simulink model "Lab2_3_sol"  (R2015b)
settings: Solver=VariableStepDiscrete  StartTime=0.0  StopTime=256*256*2  RelTol=1e-3
PreLoadFcn:
  | ImSize = 256;
undefined symbols (not defined in the file): gray
libraries: xbsIndex_r4 x32, dspsigattribs x5, visionsinks x2, visionsources x1
settings Model: Creator=arvinds  LastModifiedBy=duncanm
settings DataIOCC: SaveFormat=Array  SignalLoggingSaveFormat=ModelDataLogs
settings OptimizationCC: ExpressionDepthLimit=2147483647
settings DebuggingCC: UnderspecifiedInitializationDetection=Classic  MergeDetectMultiDrivingBlocksExec=none  SolverPrmCheckMsg=warning  FcnCallInpInsideContextMsg=EnableAllAsWarning  StateNameClashWarn=warning
settings HardwareCC: ProdBitPerPointer=32  ProdLargestAtomicFloat=None  ProdIntDivRoundTo=Undefined  ProdEndianess=Unspecified  ProdWordSize=32  ProdHWDeviceType=32-bit Generic
settings GRTTargetCC: GeneratePreprocessorConditionals=Disable all  CombineOutputUpdateFcns=off  GRTInterface=on
settings ConfigComp: CovModelRefEnable=Off  CovSFcnEnable=off

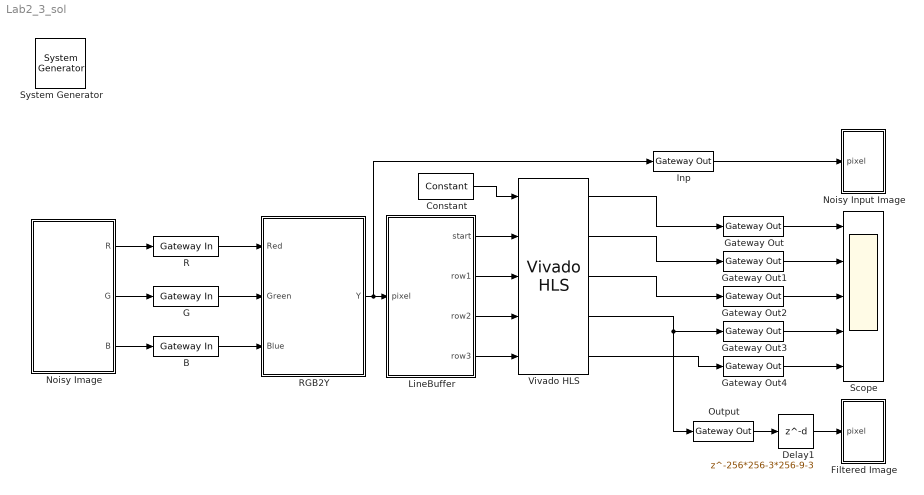
== system Lab2_3_sol ==
  " System Generator" : xbsIndex_r4/ System Generator  Tag=genX  xilinxfamily=kintex7  part=xc7k325t  speed=-3  package=fbg676  synthesis_tool=Vivado  clock_wrapper=Clock Enables  directory=./netlist  proj_type=Project Navigator  Synth_file=XST Defaults  Impl_file=ISE Defaults  testbench=off  simulink_period=1  sysclk_period=5  dcm_input_clock_period=10  incr_netlist=off  trim_vbits=Everywhere in SubSystem  dbl_ovrd=According to Block Masks  core_generation=According to Block Masks  run_coregen=off  deprecated_control=off  eval_field=0  block_type=sysgen
      settings: block_version=14.2
  B : xbsIndex_r4/Gateway In  gui_display_data_type=Fixed-point  arith_type=Unsigned  n_bits=8  bin_pt=0  preci_type=Single  exp_width=8  frac_width=24  rows=1  columns=1  quantization="Round  (unbiased: +/- Inf)"  overflow=Saturate  period=1  UseAsADC=off  ADCChannel='1'  interface=None  automatic_assignment=on  address_offset=hex2dec('00')  intf_name=''  intf_description=''  default_value=0  timing_constraint=None  locs_specified=off  LOCs={}  io_standard={}  inherit_from_input=off  hdl_port=on  dbl_ovrd=off  block_type=gatewayin
      settings: block_version=14.2
  Constant : xbsIndex_r4/Constant  const=0  gui_display_data_type=Boolean  arith_type=Boolean  n_bits=16  bin_pt=14  preci_type=Single  exp_width=8  frac_width=24  explicit_period=off  period=1  equ=P=C  opselect=C  inp2=PCIN>>17  opr=+  inp1=P  carry=CIN  dbl_ovrd=off  block_type=constant
  Delay1 : Delay  DelayLength=256*256-3*256-9-3  SampleTime=1
  Filtered Image : Subsystem
  G : xbsIndex_r4/Gateway In  gui_display_data_type=Fixed-point  arith_type=Unsigned  n_bits=8  bin_pt=0  preci_type=Single  exp_width=8  frac_width=24  rows=1  columns=1  quantization="Round  (unbiased: +/- Inf)"  overflow=Saturate  period=1  UseAsADC=off  ADCChannel='1'  interface=None  automatic_assignment=on  address_offset=hex2dec('00')  intf_name=''  intf_description=''  default_value=0  timing_constraint=None  locs_specified=off  LOCs={}  io_standard={}  inherit_from_input=off  hdl_port=on  dbl_ovrd=off  block_type=gatewayin
      settings: block_version=14.2
  Gateway Out{,1..4} (5 alike) : xbsIndex_r4/Gateway Out  inherit_from_input=off  hdl_port=on  rows=1  columns=1  UseAsDAC=off  DACChannel='1'  interface=None  automatic_assignment=on  address_offset=hex2dec('00')  intf_name=''  intf_description=''  timing_constraint=None  locs_specified=off  LOCs={}  io_standard={}  block_type=gatewayout
  Inp : xbsIndex_r4/Gateway Out  inherit_from_input=on  hdl_port=off  rows=1  columns=1  UseAsDAC=off  DACChannel='1'  interface=None  automatic_assignment=on  address_offset=hex2dec('00')  intf_name=''  intf_description=''  timing_constraint=None  locs_specified=off  LOCs={}  io_standard={}  block_type=gatewayout
      settings: block_version=14.2
  LineBuffer : Subsystem
  Noisy Image : Subsystem
  Noisy Input Image : Subsystem
  Output : xbsIndex_r4/Gateway Out  inherit_from_input=on  hdl_port=on  rows=1  columns=1  UseAsDAC=off  DACChannel='1'  interface=None  automatic_assignment=on  address_offset=hex2dec('00')  intf_name=''  intf_description=''  timing_constraint=None  locs_specified=off  LOCs={}  io_standard={}  block_type=gatewayout
      settings: block_version=14.2
  R : xbsIndex_r4/Gateway In  gui_display_data_type=Fixed-point  arith_type=Unsigned  n_bits=8  bin_pt=0  preci_type=Single  exp_width=8  frac_width=24  rows=1  columns=1  quantization="Round  (unbiased: +/- Inf)"  overflow=Saturate  period=1  UseAsADC=off  ADCChannel='1'  interface=None  automatic_assignment=on  address_offset=hex2dec('00')  intf_name=''  intf_description=''  default_value=0  timing_constraint=None  locs_specified=off  LOCs={}  io_standard={}  inherit_from_input=off  hdl_port=on  dbl_ovrd=off  block_type=gatewayin
      settings: block_version=14.2
  RGB2Y : Subsystem
  Scope : Scope  NumInputPorts=5
  Vivado HLS : xbsIndex_r4/Vivado HLS  anytable='C:/SysGen_Tutorial/Lab7/hls_project/solution1'  fast_sim=off  display_datatype=off  rate_propagation_method=Simulink system period  model_file_path=''  latency=1  block_type=hls
      settings: infoedit=This block allows including C,C++ and SystemC source files in System Generator for DSP designs.
  wires:
  Noisy Image/2(G) -> G/1
  Noisy Image/3(B) -> B/1
  R/1 -> RGB2Y/1(Red)
  G/1 -> RGB2Y/2(Green)
  B/1 -> RGB2Y/3(Blue)
  RGB2Y/1(Y) -> LineBuffer/1(pixel), Inp/1
  LineBuffer/2(row1) -> Vivado HLS/3
  LineBuffer/3(row2) -> Vivado HLS/4
  LineBuffer/4(row3) -> Vivado HLS/5
  Noisy Image/1(R) -> R/1
  Output/1 -> Delay1/1
  Inp/1 -> Noisy Input Image/1(pixel)
  Delay1/1 -> Filtered Image/1(pixel)
  Vivado HLS/4 -> Output/1, Gateway Out3/1
  Vivado HLS/1 -> Gateway Out/1
  Vivado HLS/2 -> Gateway Out1/1
  Vivado HLS/3 -> Gateway Out2/1
  Vivado HLS/5 -> Gateway Out4/1
  Gateway Out/1 -> Scope/1
  Gateway Out1/1 -> Scope/2
  Gateway Out2/1 -> Scope/3
  Gateway Out3/1 -> Scope/4
  Gateway Out4/1 -> Scope/5
  LineBuffer/1(start) -> Vivado HLS/2
  Constant/1 -> Vivado HLS/1

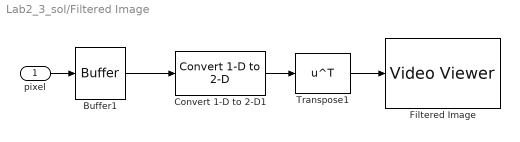
== system Lab2_3_sol/Filtered Image ==
  pixel : Inport
  Buffer1 : Buffer  N=ImSize*ImSize  TreatMby1Signals=One channel
  Convert 1-D to 2-D1 : dspsigattribs/Convert 1-D to 2-D  M=ImSize  N=ImSize  frameBasedOut=off
  Filtered Image : visionsinks/Video Viewer  inputType=Obsolete7b  imagePorts=One multidimensional signal  useColorMap=off  colormapValue=gray(256)  specRange=off  minInputVal=0  maxInputVal=255  FigPos=[721 702.8 408 300]  AxisZoom=on  trueSizedOnce=off  OpenAtMdlStart=on  DefaultConfigurationName=vipscopes.VideoViewerScopeCfg
  Transpose1 : Math  Operator=transpose  SaturateOnIntegerOverflow=on
  wires:
  Buffer1/1 -> Convert 1-D to 2-D1/1
  Convert 1-D to 2-D1/1 -> Transpose1/1
  pixel/1 -> Buffer1/1
  Transpose1/1 -> Filtered Image/1

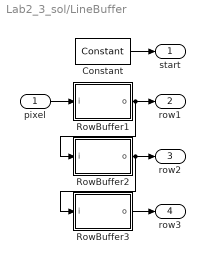
== system Lab2_3_sol/LineBuffer ==
  pixel : Inport
  Constant : xbsIndex_r4/Constant  const=1  gui_display_data_type=Boolean  arith_type=Boolean  n_bits=16  bin_pt=14  preci_type=Single  exp_width=8  frac_width=24  explicit_period=off  period=1  equ=P=C  opselect=C  inp2=PCIN>>17  opr=+  inp1=P  carry=CIN  dbl_ovrd=off  block_type=constant
  RowBuffer1 : Subsystem  mask(Virtex2 Line Buffer){buf_depth=ImSize, cst=1}
      mask prompts: buf_depth "Buffer Depth"; cst "Sample Period"
      mask help: The Xilinx Virtex2 Line Buffer reference block delayes a sequential stream of pixels by the specified buffer depth. It is optimized for the Virtex2 family since it uses the Read Before Write option on the underlying Single Port RAM block.
      mask init:
      | str = sprintf('-%d',buf_depth);
      | [bg,fg] = xlcmap('XBlock',0);
      | iPos = get_param(gcb,'Position');
      | iWidth=iPos(3)-iPos(1); iHeight=iPos(4)-iPos(2);
      | iCx=iWidth/2;
      | iCy=iHeight/2;
      | [logoX, logoY] = xlogo(iPos);
      mask Help: eval('');xlDoc('-book','sysgen','-topic','Virtex2_Line_Buffer');
      mask Display:
      | patch([0 iWidth iWidth 0],[0 0 iHeight iHeight] , bg);
      | patch(logoX,logoY , fg);
      | text(iCx-6,iCy,'z');
      | text(iCx,iCy+4,str);
      | plot([0 0 iWidth iWidth 0], [0 iHeight iHeight 0 0]);
  RowBuffer2 : Subsystem  mask(Virtex2 Line Buffer){buf_depth=ImSize, cst=1}
      mask prompts: buf_depth "Buffer Depth"; cst "Sample Period"
      mask help: The Xilinx Virtex2 Line Buffer reference block delayes a sequential stream of pixels by the specified buffer depth. It is optimized for the Virtex2 family since it uses the Read Before Write option on the underlying Single Port RAM block.
      mask init: same as Lab2_3_sol/LineBuffer/RowBuffer1
      mask Help: eval('');xlDoc('-book','sysgen','-topic','Virtex2_Line_Buffer');
      mask Display:
      | patch([0 iWidth iWidth 0],[0 0 iHeight iHeight] , bg);
      | patch(logoX,logoY , fg);
      | text(iCx-6,iCy,'z');
      | text(iCx,iCy+4,str);
      | plot([0 0 iWidth iWidth 0], [0 iHeight iHeight 0 0]);
  RowBuffer3 : Subsystem  mask(Virtex2 Line Buffer){buf_depth=ImSize, cst=1}
      mask prompts: buf_depth "Buffer Depth"; cst "Sample Period"
      mask help: The Xilinx Virtex2 Line Buffer reference block delayes a sequential stream of pixels by the specified buffer depth. It is optimized for the Virtex2 family since it uses the Read Before Write option on the underlying Single Port RAM block.
      mask init: same as Lab2_3_sol/LineBuffer/RowBuffer1
      mask Help: eval('');xlDoc('-book','sysgen','-topic','Virtex2_Line_Buffer');
      mask Display:
      | patch([0 iWidth iWidth 0],[0 0 iHeight iHeight] , bg);
      | patch(logoX,logoY , fg);
      | text(iCx-6,iCy,'z');
      | text(iCx,iCy+4,str);
      | plot([0 0 iWidth iWidth 0], [0 iHeight iHeight 0 0]);
  start : Outport
  row1 : Outport  Port=2
  row2 : Outport  Port=3
  row3 : Outport  Port=4
  wires:
  RowBuffer1/1(o) -> RowBuffer2/1(i), row1/1
  RowBuffer2/1(o) -> RowBuffer3/1(i), row2/1
  pixel/1 -> RowBuffer1/1(i)
  RowBuffer3/1(o) -> row3/1
  Constant/1 -> start/1

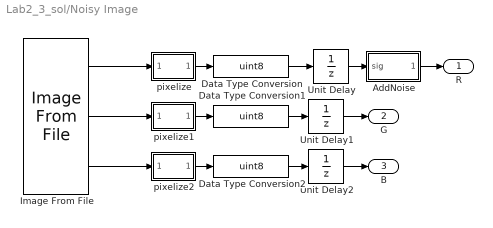
== system Lab2_3_sol/Noisy Image ==
  AddNoise : Subsystem
  Data Type Conversion : DataTypeConversion  OutDataTypeStr=uint8
  Data Type Conversion1 : DataTypeConversion  OutDataTypeStr=uint8
  Data Type Conversion2 : DataTypeConversion  OutDataTypeStr=uint8
  Image From File : visionsources/Image From File  Tag=vipblks_nd  FileName=C:\SysGen_Tutorial\Lab7\lena.jpg  imagePorts=Separate color signals  Ts=ImSize*ImSize  ImageDataType=uint8  Signed=on  WordLength=16  sdImageDataType=uint(8)  FractionLengthMode=User-defined  FractionLength=15  OutPortLabels=R|G|B
  Unit Delay : UnitDelay  SampleTime=-1
  Unit Delay1 : UnitDelay  SampleTime=-1
  Unit Delay2 : UnitDelay  SampleTime=-1
  pixelize : Subsystem
  pixelize1 : Subsystem
  pixelize2 : Subsystem
  R : Outport
  G : Outport  Port=2
  B : Outport  Port=3
  wires:
  Image From File/1 -> pixelize/1(In1)
  Data Type Conversion/1 -> Unit Delay/1
  pixelize/1(Out1) -> Data Type Conversion/1
  Data Type Conversion1/1 -> Unit Delay1/1
  pixelize1/1(Out1) -> Data Type Conversion1/1
  Image From File/2 -> pixelize1/1(In1)
  Data Type Conversion2/1 -> Unit Delay2/1
  pixelize2/1(Out1) -> Data Type Conversion2/1
  Image From File/3 -> pixelize2/1(In1)
  Unit Delay/1 -> AddNoise/1(sig)
  AddNoise/1(noise_sig) -> R/1
  Unit Delay1/1 -> G/1
  Unit Delay2/1 -> B/1

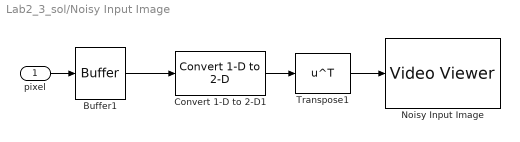
== system Lab2_3_sol/Noisy Input Image ==
  pixel : Inport
  Buffer1 : Buffer  N=ImSize*ImSize  TreatMby1Signals=One channel
  Convert 1-D to 2-D1 : dspsigattribs/Convert 1-D to 2-D  M=ImSize  N=ImSize  frameBasedOut=off
  Noisy Input Image : visionsinks/Video Viewer  inputType=Obsolete7b  imagePorts=One multidimensional signal  useColorMap=off  colormapValue=gray(256)  specRange=off  minInputVal=0  maxInputVal=255  FigPos=[291.4 702.8 409.6 300]  AxisZoom=on  trueSizedOnce=off  OpenAtMdlStart=on  DefaultConfigurationName=vipscopes.VideoViewerScopeCfg
  Transpose1 : Math  Operator=transpose  SaturateOnIntegerOverflow=on
  wires:
  Buffer1/1 -> Convert 1-D to 2-D1/1
  Convert 1-D to 2-D1/1 -> Transpose1/1
  pixel/1 -> Buffer1/1
  Transpose1/1 -> Noisy Input Image/1

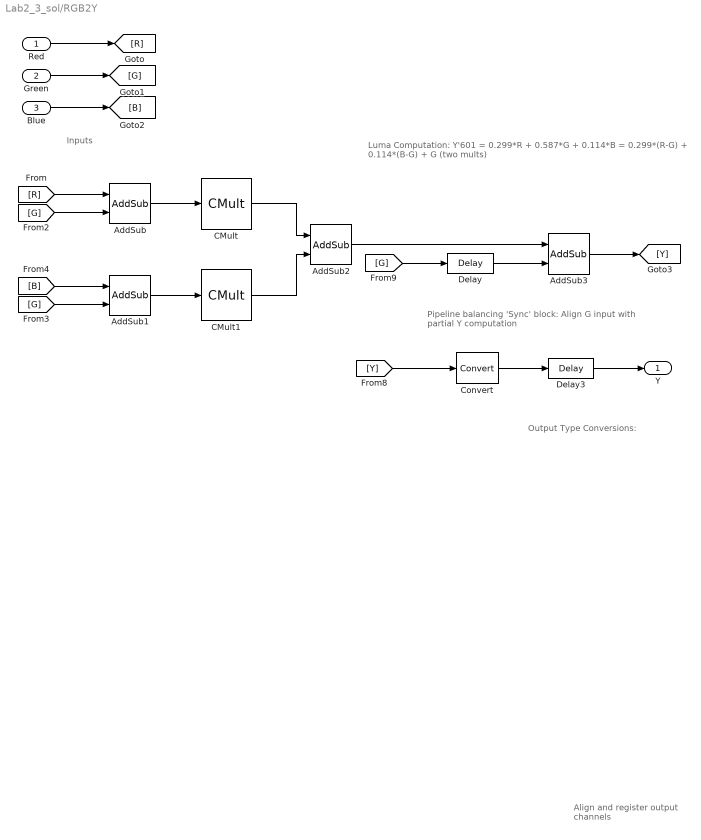
== system Lab2_3_sol/RGB2Y ==
  note: Luma Computation:
      |
      |  Y'601 = 0.299*R + 0.587*G + 0.114*B
      |           = 0.299*(R-G) + 0.114*(B-G) + G   (two mults)
  note: Inputs
  note: Pipeline balancing 'Sync' block:
      | Align G input with partial Y computation
  note: Align and register
      | output channels
  note: Output Type Conversions:
  Red : Inport
  Green : Inport  Port=2
  Blue : Inport  Port=3
  AddSub : xbsIndex_r4/AddSub  mode=Subtraction  use_carryin=off  use_carryout=off  en=off  latency=1  precision=Full  arith_type=Unsigned  n_bits=8  bin_pt=2  quantization=Truncate  overflow=Wrap  use_behavioral_HDL=off  hw_selection=Fabric  pipelined=off  use_rpm=off  dbl_ovrd=off  block_type=addsub
      settings: xl_area=[6 11 0 11 0 0 0]  block_version=VER_STRING_GOES_HERE
  AddSub1 : xbsIndex_r4/AddSub  mode=Subtraction  use_carryin=off  use_carryout=off  en=off  latency=1  precision=Full  arith_type=Unsigned  n_bits=8  bin_pt=2  quantization=Truncate  overflow=Wrap  use_behavioral_HDL=off  hw_selection=Fabric  pipelined=off  use_rpm=off  dbl_ovrd=off  block_type=addsub
      settings: xl_area=[6 11 0 11 0 0 0]  block_version=VER_STRING_GOES_HERE
  AddSub2 : xbsIndex_r4/AddSub  mode=Addition  use_carryin=off  use_carryout=off  en=off  latency=1  precision=Full  arith_type=Unsigned  n_bits=8  bin_pt=2  quantization=Truncate  overflow=Wrap  use_behavioral_HDL=off  hw_selection=Fabric  pipelined=off  use_rpm=off  dbl_ovrd=off  block_type=addsub
      settings: xl_area=[13 24 0 24 0 0 0]  block_version=VER_STRING_GOES_HERE
  AddSub3 : xbsIndex_r4/AddSub  mode=Addition  use_carryin=off  use_carryout=off  en=off  latency=1  precision=User Defined  arith_type="Signed  (2's comp)"  n_bits=10  bin_pt=0  quantization="Round  (unbiased: +/- Inf)"  overflow=Saturate  use_behavioral_HDL=off  hw_selection=Fabric  pipelined=off  use_rpm=off  dbl_ovrd=off  block_type=addsub
      settings: xl_area=[24 10 0 45 0 0 0]  block_version=VER_STRING_GOES_HERE
  CMult : xbsIndex_r4/CMult  const=0.299  gui_display_data_type=Fixed-point  const_n_bits=12  const_bin_pt=12  float_type=Single  exp_bits=8  fraction_bits=24  en=off  latency=3  precision=Full  arith_type="Signed  (2's comp)"  n_bits=8  bin_pt=2  quantization="Round  (unbiased: +/- Inf)"  overflow=Wrap  use_behavioral_HDL=off  mem_type=Distributed RAM  pipeline=off  use_rpm=off  placement_style=Triangular Packing  dbl_ovrd=off  block_type=cmult
      settings: xl_area=[51 100 0 76 0 0 0]  block_version=VER_STRING_GOES_HERE
  CMult1 : xbsIndex_r4/CMult  const=0.114  gui_display_data_type=Fixed-point  const_n_bits=12  const_bin_pt=12  float_type=Single  exp_bits=8  fraction_bits=24  en=off  latency=3  precision=Full  arith_type="Signed  (2's comp)"  n_bits=8  bin_pt=2  quantization="Round  (unbiased: +/- Inf)"  overflow=Wrap  use_behavioral_HDL=off  mem_type=Distributed RAM  pipeline=off  use_rpm=off  placement_style=Triangular Packing  dbl_ovrd=off  block_type=cmult
      settings: xl_area=[45 88 0 66 0 0 0]  block_version=VER_STRING_GOES_HERE
  Convert : xbsIndex_r4/Convert  gui_display_data_type=Fixed-point  arith_type=Unsigned  n_bits=8  bin_pt=0  float_type=Single  exp_bits=8  fraction_bits=24  quantization="Round  (unbiased: +/- Inf)"  overflow=Saturate  en=off  latency=0  pipeline=off  dbl_ovrd=off  block_type=convert
      settings: xl_area=[0 0 0 0 0 0 0]  block_version=VER_STRING_GOES_HERE
  Delay : xbsIndex_r4/Delay  rst=off  infoeditControl=Selection of Reset will increase slice count due to use of real FFs and instead of SRLs  en=off  latency=5  reg_retiming=off  dbl_ovrd=off  block_type=delay
      settings: infoedit="Delay line having  configurable length.<P><P>Hardware notes: A delay line is a chain, each link of which is an SRL16 followed by a flip-flop. If register retiming is enabled, the delay line is a chain of flip-flops."  xl_area=[0, 0, 0, 0, 0, 0, 0]  block_version=VER_STRING_GOES_HERE
  Delay3 : xbsIndex_r4/Delay  rst=off  infoeditControl=Selection of Reset will increase slice count due to use of real FFs and instead of SRLs  en=off  latency=5  reg_retiming=off  dbl_ovrd=off  block_type=delay
      settings: infoedit="Delay line having  configurable length.<P><P>Hardware notes: A delay line is a chain, each link of which is an SRL16 followed by a flip-flop. If register retiming is enabled, the delay line is a chain of flip-flops."  xl_area=[0, 0, 0, 0, 0, 0, 0]  block_version=VER_STRING_GOES_HERE
  Y : Outport
  wires:
  [G] -> AddSub/2
  [G] -> Delay/1
  Delay/1 -> AddSub3/2
  AddSub3/1 -> [Y]
  [B] -> AddSub1/1
  [G] -> AddSub1/2
  [R] -> AddSub/1
  Blue/1 -> [B]
  Green/1 -> [G]
  Red/1 -> [R]
  [Y] -> Convert/1
  CMult/1 -> AddSub2/1
  CMult1/1 -> AddSub2/2
  AddSub/1 -> CMult/1
  AddSub1/1 -> CMult1/1
  AddSub2/1 -> AddSub3/1
  Delay3/1 -> Y/1
  Convert/1 -> Delay3/1

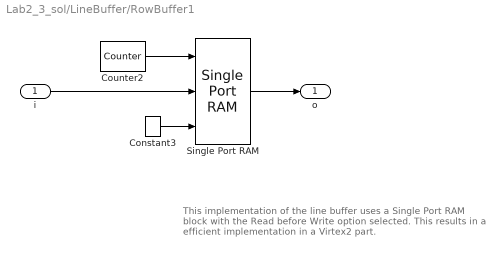
== system Lab2_3_sol/LineBuffer/RowBuffer1 ==
  note: This implementation of the line buffer uses a
      |  Single Port RAM block with the Read before Write
      | option selected.  This results in a efficient
      | implementation in a Virtex2 part.
  i : Inport
  Constant3 : xbsIndex_r4/Constant  const=1  gui_display_data_type=Fixed-point  arith_type=Boolean  n_bits=1  bin_pt=0  preci_type=Single  exp_width=8  frac_width=24  explicit_period=on  period=cst  equ=P=C  opselect=C  inp2=PCIN>>17  opr=+  inp1=P  carry=CIN  dbl_ovrd=off  block_type=constant
      settings: block_version=VER_STRING_GOES_HERE
  Counter2 : xbsIndex_r4/Counter  cnt_type=Count Limited  cnt_to=buf_depth -2  operation=Up  start_count=0  cnt_by_val=1  arith_type=Unsigned  n_bits=ceil(log2(buf_depth-1))  bin_pt=0  load_pin=off  rst=off  en=off  explicit_period=on  period=cst  use_behavioral_HDL=off  implementation=Fabric  dbl_ovrd=off  block_type=counter
      settings: infoedit="Configurable up, down and up/down counter.<P><P>Hardware notes: Free running counters are the least expensive in hardware.  A count limited counter is implemented by combining a counter with a comparator."  xl_area=[7 10 0 13 0 0 0]  block_version=VER_STRING_GOES_HERE
  Single Port RAM : xbsIndex_r4/Single Port RAM  depth=buf_depth-1  initVector=0  distributed_mem=Block RAM  write_mode=Read Before Write  rst=off  init_reg=0  en=off  latency=1  optimize=Area  dbl_ovrd=off  block_type=spram
      settings: xl_area=[0 0 1 0 0 0 0]  block_version=8.2
  o : Outport
  wires:
  Constant3/1 -> Single Port RAM/3
  Single Port RAM/1 -> o/1
  i/1 -> Single Port RAM/2
  Counter2/1 -> Single Port RAM/1

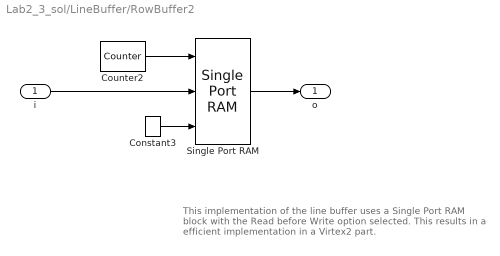
== system Lab2_3_sol/LineBuffer/RowBuffer2 ==
  note: This implementation of the line buffer uses a
      |  Single Port RAM block with the Read before Write
      | option selected.  This results in a efficient
      | implementation in a Virtex2 part.
  i : Inport
  Constant3 : xbsIndex_r4/Constant  const=1  gui_display_data_type=Fixed-point  arith_type=Boolean  n_bits=1  bin_pt=0  preci_type=Single  exp_width=8  frac_width=24  explicit_period=on  period=cst  equ=P=C  opselect=C  inp2=PCIN>>17  opr=+  inp1=P  carry=CIN  dbl_ovrd=off  block_type=constant
      settings: block_version=VER_STRING_GOES_HERE
  Counter2 : xbsIndex_r4/Counter  cnt_type=Count Limited  cnt_to=buf_depth -2  operation=Up  start_count=0  cnt_by_val=1  arith_type=Unsigned  n_bits=ceil(log2(buf_depth-1))  bin_pt=0  load_pin=off  rst=off  en=off  explicit_period=on  period=cst  use_behavioral_HDL=off  implementation=Fabric  dbl_ovrd=off  block_type=counter
      settings: infoedit="Configurable up, down and up/down counter.<P><P>Hardware notes: Free running counters are the least expensive in hardware.  A count limited counter is implemented by combining a counter with a comparator."  xl_area=[7 10 0 13 0 0 0]  block_version=VER_STRING_GOES_HERE
  Single Port RAM : xbsIndex_r4/Single Port RAM  depth=buf_depth-1  initVector=0  distributed_mem=Block RAM  write_mode=Read Before Write  rst=off  init_reg=0  en=off  latency=1  optimize=Area  dbl_ovrd=off  block_type=spram
      settings: xl_area=[0 0 1 0 0 0 0]  block_version=8.2
  o : Outport
  wires:
  Counter2/1 -> Single Port RAM/1
  i/1 -> Single Port RAM/2
  Single Port RAM/1 -> o/1
  Constant3/1 -> Single Port RAM/3

== system Lab2_3_sol/LineBuffer/RowBuffer3 ==
  note: This implementation of the line buffer uses a
      |  Single Port RAM block with the Read before Write
      | option selected.  This results in a efficient
      | implementation in a Virtex2 part.
  i : Inport
  Constant3 : xbsIndex_r4/Constant  const=1  gui_display_data_type=Fixed-point  arith_type=Boolean  n_bits=1  bin_pt=0  preci_type=Single  exp_width=8  frac_width=24  explicit_period=on  period=cst  equ=P=C  opselect=C  inp2=PCIN>>17  opr=+  inp1=P  carry=CIN  dbl_ovrd=off  block_type=constant
      settings: block_version=VER_STRING_GOES_HERE
  Counter2 : xbsIndex_r4/Counter  cnt_type=Count Limited  cnt_to=buf_depth -2  operation=Up  start_count=0  cnt_by_val=1  arith_type=Unsigned  n_bits=ceil(log2(buf_depth-1))  bin_pt=0  load_pin=off  rst=off  en=off  explicit_period=on  period=cst  use_behavioral_HDL=off  implementation=Fabric  dbl_ovrd=off  block_type=counter
      settings: infoedit="Configurable up, down and up/down counter.<P><P>Hardware notes: Free running counters are the least expensive in hardware.  A count limited counter is implemented by combining a counter with a comparator."  xl_area=[7 10 0 13 0 0 0]  block_version=VER_STRING_GOES_HERE
  Single Port RAM : xbsIndex_r4/Single Port RAM  depth=buf_depth-1  initVector=0  distributed_mem=Block RAM  write_mode=Read Before Write  rst=off  init_reg=0  en=off  latency=1  optimize=Area  dbl_ovrd=off  block_type=spram
      settings: xl_area=[0 0 1 0 0 0 0]  block_version=8.2
  o : Outport
  wires:
  Constant3/1 -> Single Port RAM/3
  Single Port RAM/1 -> o/1
  i/1 -> Single Port RAM/2
  Counter2/1 -> Single Port RAM/1

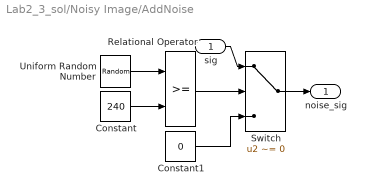
== system Lab2_3_sol/Noisy Image/AddNoise ==
  sig : Inport
  Constant : Constant  Value=240
  Constant1 : Constant  Value=0
  Relational Operator : RelationalOperator  OutDataTypeStr=boolean  SampleTime=1
  Switch : Switch  Criteria=u2 ~= 0  SampleTime=1
  Uniform Random Number : UniformRandomNumber  Minimum=0  Maximum=255  SampleTime=1
  noise_sig : Outport
  wires:
  Uniform Random Number/1 -> Relational Operator/1
  Relational Operator/1 -> Switch/2
  Constant/1 -> Relational Operator/2
  Constant1/1 -> Switch/3
  sig/1 -> Switch/1
  Switch/1 -> noise_sig/1

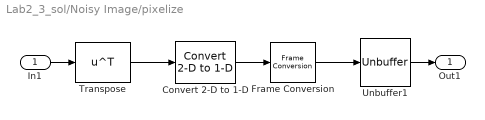
== system Lab2_3_sol/Noisy Image/pixelize ==
  In1 : Inport
  Convert 2-D to 1-D : dspsigattribs/Convert 2-D to 1-D
  Frame Conversion : FrameConversion  InheritSamplingMode=off
  Transpose : Math  Operator=transpose  SaturateOnIntegerOverflow=on
  Unbuffer1 : Unbuffer  SampleBasedProcessing=Same as frame based
  Out1 : Outport
  wires:
  Convert 2-D to 1-D/1 -> Frame Conversion/1
  Frame Conversion/1 -> Unbuffer1/1
  Transpose/1 -> Convert 2-D to 1-D/1
  In1/1 -> Transpose/1
  Unbuffer1/1 -> Out1/1

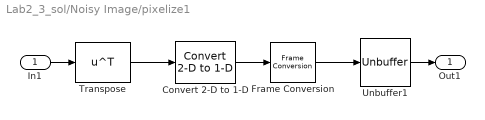
== system Lab2_3_sol/Noisy Image/pixelize1 ==
  In1 : Inport
  Convert 2-D to 1-D : dspsigattribs/Convert 2-D to 1-D
  Frame Conversion : FrameConversion  InheritSamplingMode=off
  Transpose : Math  Operator=transpose  SaturateOnIntegerOverflow=on
  Unbuffer1 : Unbuffer  SampleBasedProcessing=Same as frame based
  Out1 : Outport
  wires:
  Unbuffer1/1 -> Out1/1
  In1/1 -> Transpose/1
  Transpose/1 -> Convert 2-D to 1-D/1
  Frame Conversion/1 -> Unbuffer1/1
  Convert 2-D to 1-D/1 -> Frame Conversion/1

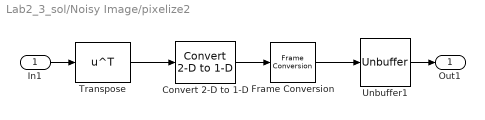
== system Lab2_3_sol/Noisy Image/pixelize2 ==
  In1 : Inport
  Convert 2-D to 1-D : dspsigattribs/Convert 2-D to 1-D
  Frame Conversion : FrameConversion  InheritSamplingMode=off
  Transpose : Math  Operator=transpose  SaturateOnIntegerOverflow=on
  Unbuffer1 : Unbuffer  SampleBasedProcessing=Same as frame based
  Out1 : Outport
  wires:
  Convert 2-D to 1-D/1 -> Frame Conversion/1
  Frame Conversion/1 -> Unbuffer1/1
  Transpose/1 -> Convert 2-D to 1-D/1
  In1/1 -> Transpose/1
  Unbuffer1/1 -> Out1/1
